simulink model "HW4Model"  (R2022b)
settings: Solver=VariableStepAuto  StartTime=0.0  StopTime=10.0  RelTol=1e-3
undefined symbols (not defined in the file): sat, trigger
settings Model: Creator=gagandeepthapar  LastModifiedBy=gagandeepthapar

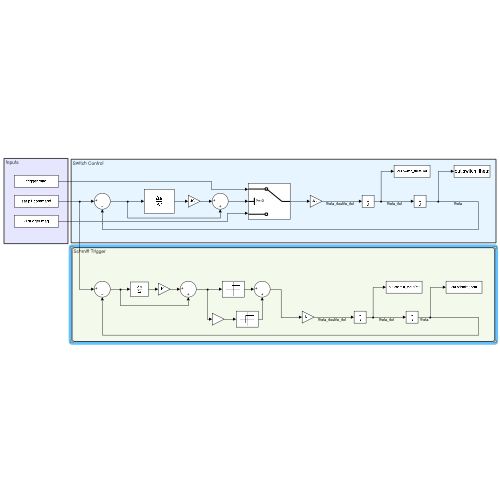
[thumbnail: Simulink's stored preview of the top-level diagram]
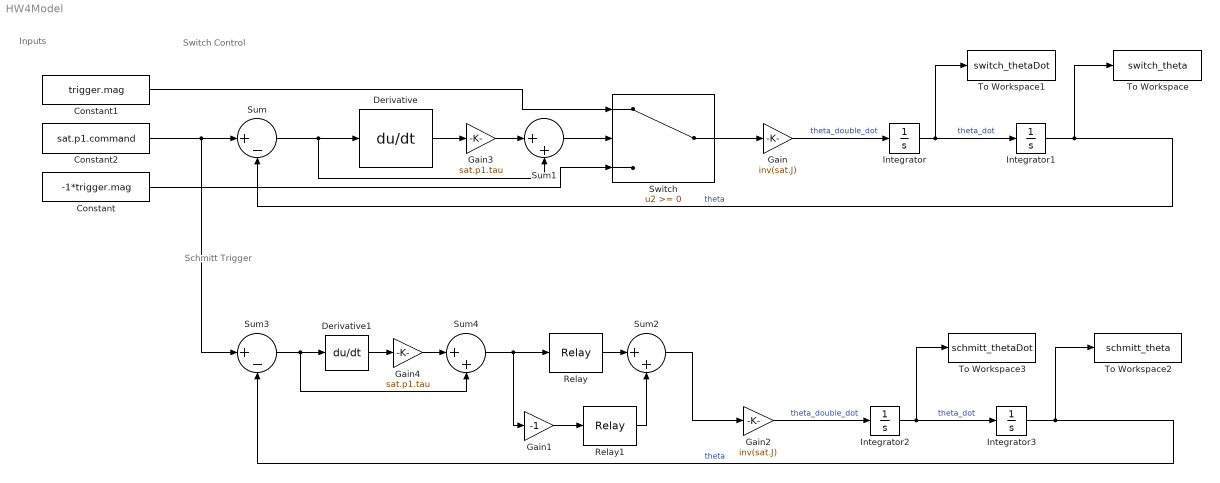
== system HW4Model ==
  note: Schmitt Trigger
  note: Switch Control
  note: Inputs
  Constant : Constant  Value=-1*trigger.mag
  Constant1 : Constant  Value=trigger.mag
  Constant2 : Constant  Value=sat.p1.command
  Derivative : Derivative
  Derivative1 : Derivative
  Gain : Gain  Gain=inv(sat.J)
  Gain1 : Gain  Gain=-1
  Gain2 : Gain  Gain=inv(sat.J)
  Gain3 : Gain  Gain=sat.p1.tau
  Gain4 : Gain  Gain=sat.p1.tau
  Integrator : Integrator
  Integrator1 : Integrator  InitialCondition=sat.p1.initial
  Integrator2 : Integrator
  Integrator3 : Integrator  InitialCondition=sat.p1.initial
  Relay : Relay  OnSwitchValue=trigger.delOn  OffSwitchValue=trigger.delOff  OnOutputValue=trigger.mag
  Relay1 : Relay  OnSwitchValue=trigger.delOn  OffSwitchValue=trigger.delOff  OnOutputValue=-1*trigger.mag
  Sum : Sum  Inputs=|+-
  Sum1 : Sum  Inputs=|++
  Sum2 : Sum  Inputs=|++
  Sum3 : Sum  Inputs=|+-
  Sum4 : Sum  Inputs=|++
  Switch : Switch  ZeroCross=off  SaturateOnIntegerOverflow=off  InputSameDT=off
  To Workspace : ToWorkspace  VariableName=switch_theta  SampleTime=-1
      settings: Save2DSignal=2-D array (concatenate along first dimension)
  To Workspace1 : ToWorkspace  VariableName=switch_thetaDot  SampleTime=-1
      settings: Save2DSignal=2-D array (concatenate along first dimension)
  To Workspace2 : ToWorkspace  VariableName=schmitt_theta  SampleTime=-1
      settings: Save2DSignal=2-D array (concatenate along first dimension)
  To Workspace3 : ToWorkspace  VariableName=schmitt_thetaDot  SampleTime=-1
      settings: Save2DSignal=2-D array (concatenate along first dimension)
  wires:
  Integrator1/1 -> To Workspace/1, Sum/2  "theta"
  Integrator/1 -> To Workspace1/1, Integrator1/1  "theta_dot"
  Switch/1 -> Gain/1
  Sum/1 -> Sum1/2, Derivative/1
  Gain/1 -> Integrator/1  "theta_double_dot"
  Sum1/1 -> Switch/2
  Constant/1 -> Switch/3
  Constant1/1 -> Switch/1
  Constant2/1 -> Sum3/1, Sum/1
  Gain1/1 -> Relay1/1
  Relay/1 -> Sum2/1
  Relay1/1 -> Sum2/2
  Gain2/1 -> Integrator2/1  "theta_double_dot"
  Integrator2/1 -> To Workspace3/1, Integrator3/1  "theta_dot"
  Integrator3/1 -> To Workspace2/1, Sum3/2  "theta"
  Sum2/1 -> Gain2/1
  Sum4/1 -> Gain1/1, Relay/1
  Sum3/1 -> Derivative1/1, Sum4/2
  Gain3/1 -> Sum1/1
  Derivative/1 -> Gain3/1
  Derivative1/1 -> Gain4/1
  Gain4/1 -> Sum4/1
